simulink model "chris_3R_hsv_all_primitives_fixed_vortex"  (R2024b)
settings: Solver=FixedStepDiscrete  StartTime=0.0  StopTime=10  FixedStep=0.1  MaxStep=0.1  RelTol=1e-3
libraries: neural x102, realtime_pacer_lib x1, simulink x1
(part 6 of 6)

== matlab function chris_3R_hsv_all_primitives_fixed_vortex/all_bot_version2/sat_post_processor1 ==
  data: data output; data_raw input
function data = data_normalizing(data_raw)

data = (data_raw*2)-1;


end

== matlab function chris_3R_hsv_all_primitives_fixed_vortex/vector2scalar _avg_direction_only/Cluster Velocities to Cartesian Velocities ==
  data: fwdkin input; xc_err input; x1 output; zc_err input; thC_err input; a_err input; b_err input; C_err input; z1 output; th1 output; x2 output; z2 output; th2 output; x3 output; z3 output; th3 output
function [x1, z1,th1, x2,z2,th2, x3,z3, th3] = InverseJabobian(fwdkin, xc_err, zc_err, thC_err, a_err, b_err, C_err)
%% Unpacking the information from fwd_kin
p = fwdkin(1);
q = fwdkin(2);
beta = fwdkin(3);
xc = fwdkin(4);
yc = fwdkin(5);
theta_c = fwdkin(6);
yc_err = zc_err;
theta_c_err = thC_err;
p_err = a_err;
q_err = b_err;
beta_err = C_err;
%% Inverse Kinematics
  % Calculate x1, y1, and theta1 (Equations 12, 13, and 14)
r = sqrt((q + p*cos(beta))^2 + (p*sin(beta))^2);
  
x1 = xc + (1/3)*r*sin(theta_c);
y1 = yc + (1/3)*r*cos(theta_c);
%theta1 = phi1 - theta_c;
% Calculate x2, y2, and theta2 (Equations 15, 16, and 17)
x2 = xc + (1/3)*r*sin(theta_c) - p*sin(beta/2 + theta_c);
y2 = yc + (1/3)*r*cos(theta_c) - p*cos(beta/2 + theta_c);
%theta2 = phi2 - theta_c;
% Calculate x3, y3, and theta3 (Equations 18, 19, and 20)
x3 = xc + (1/3)*r*sin(theta_c) + q*sin(beta/2 - theta_c);
y3 = yc + (1/3)*r*cos(theta_c) - q*cos(beta/2 - theta_c);
%theta3 = phi3 - theta_c;
%% Now to take the partial derivates
% syms p q beta xc yc theta_c p_err q_err beta_err xc_err yc_err theta_c_err
% 
% % Define the equations
% eqs = [
%   xc + (1/3)*(sqrt((q + p*cos(beta))^2 + (p*sin(beta))^2))*sin(theta_c); % x1
%   yc + (1/3)*(sqrt((q + p*cos(beta))^2 + (p*sin(beta))^2))*cos(theta_c); % y1
%   xc + (1/3)*(sqrt((q + p*cos(beta))^2 + (p*sin(beta))^2))*sin(theta_c) - p*sin(beta/2 + theta_c); % x2
%   yc + (1/3)*(sqrt((q + p*cos(beta))^2 + (p*sin(beta))^2))*cos(theta_c) - p*cos(beta/2 + theta_c); % y2
%   xc + (1/3)*(sqrt((q + p*cos(beta))^2 + (p*sin(beta))^2))*sin(theta_c) + q*sin(beta/2 - theta_c); % x3
%   yc + (1/3)*(sqrt((q + p*cos(beta))^2 + (p*sin(beta))^2))*cos(theta_c) - q*cos(beta/2 - theta_c)  % y3
% ];
% 
% % Define the variables for differentiation
% vars = [p, q, beta, xc, yc, theta_c];
% 
% % Define the errors
% errs = [p_err, q_err, beta_err, xc_err, yc_err, theta_c_err];
% 
% % Initialize an array to store the sums (as symbolic)
% sums = sym(zeros(length(eqs), 1));
% 
% % Loop through equations and variables
% for i = 1:length(eqs)
%   for j = 1:length(vars)
%     derivative = diff(eqs(i), vars(j));
%     sums(i) = sums(i) + derivative * errs(j);
%   end
% end
% 
% % Display the results
% disp(simplify(sums(1)))
% disp(simplify(sums(2)))
% disp(simplify(sums(3)))
% disp(simplify(sums(4)))
% disp(simplify(sums(5)))
% disp(simplify(sums(6)))
%% Now to sum it all up
x1 =(3*xc_err*(p^2 + 2*cos(beta)*p*q + q^2)^(1/2) + p*p_err*sin(theta_c) + q*q_err*sin(theta_c) + p^2*theta_c_err*cos(theta_c) + q^2*theta_c_err*cos(theta_c) + p*q_err*cos(beta)*sin(theta_c) + p_err*q*cos(beta)*sin(theta_c) + 2*p*q*theta_c_err*cos(beta)*cos(theta_c) - beta_err*p*q*sin(beta)*sin(theta_c))/(3*(p^2 + 2*cos(beta)*p*q + q^2)^(1/2));
 
z1 = (3*yc_err*(p^2 + 2*cos(beta)*p*q + q^2)^(1/2) + p*p_err*cos(theta_c) + q*q_err*cos(theta_c) - p^2*theta_c_err*sin(theta_c) - q^2*theta_c_err*sin(theta_c) + p*q_err*cos(beta)*cos(theta_c) + p_err*q*cos(beta)*cos(theta_c) - beta_err*p*q*sin(beta)*cos(theta_c) - 2*p*q*theta_c_err*cos(beta)*sin(theta_c))/(3*(p^2 + 2*cos(beta)*p*q + q^2)^(1/2));
 
x2 = xc_err - p_err*(sin(beta/2 + theta_c) - (sin(theta_c)*(p + q*cos(beta)))/(3*(p^2 + 2*cos(beta)*p*q + q^2)^(1/2))) - beta_err*((p*cos(beta/2 + theta_c))/2 + (p*q*sin(beta)*sin(theta_c))/(3*(p^2 + 2*cos(beta)*p*q + q^2)^(1/2))) + theta_c_err*((cos(theta_c)*(p^2 + 2*cos(beta)*p*q + q^2)^(1/2))/3 - p*cos(beta/2 + theta_c)) + (q_err*sin(theta_c)*(q + p*cos(beta)))/(3*(p^2 + 2*cos(beta)*p*q + q^2)^(1/2));
 
z2 = yc_err - p_err*(cos(beta/2 + theta_c) - (cos(theta_c)*(p + q*cos(beta)))/(3*(p^2 + 2*cos(beta)*p*q + q^2)^(1/2))) + beta_err*((p*sin(beta/2 + theta_c))/2 - (p*q*sin(beta)*cos(theta_c))/(3*(p^2 + 2*cos(beta)*p*q + q^2)^(1/2))) - (theta_c_err*sin(theta_c)*(p^2 + 2*cos(beta)*p*q + q^2)^(1/2))/3 + p*theta_c_err*sin(beta/2 + theta_c) + (q_err*cos(theta_c)*(q + p*cos(beta)))/(3*(p^2 + 2*cos(beta)*p*q + q^2)^(1/2));
 
x3 = xc_err + q_err*(sin(beta/2 - theta_c) + (sin(theta_c)*(q + p*cos(beta)))/(3*(p^2 + 2*cos(beta)*p*q + q^2)^(1/2))) + beta_err*((q*cos(beta/2 - theta_c))/2 - (p*q*sin(beta)*sin(theta_c))/(3*(p^2 + 2*cos(beta)*p*q + q^2)^(1/2))) + (theta_c_err*cos(theta_c)*(p^2 + 2*cos(beta)*p*q + q^2)^(1/2))/3 - q*theta_c_err*cos(beta/2 - theta_c) + (p_err*sin(theta_c)*(p + q*cos(beta)))/(3*(p^2 + 2*cos(beta)*p*q + q^2)^(1/2));
 
z3 = yc_err - theta_c_err*(q*sin(beta/2 - theta_c) + (sin(theta_c)*(p^2 + 2*cos(beta)*p*q + q^2)^(1/2))/3) - q_err*(cos(beta/2 - theta_c) - (cos(theta_c)*(q + p*cos(beta)))/(3*(p^2 + 2*cos(beta)*p*q + q^2)^(1/2))) + beta_err*((q*sin(beta/2 - theta_c))/2 - (p*q*sin(beta)*cos(theta_c))/(3*(p^2 + 2*cos(beta)*p*q + q^2)^(1/2))) + (p_err*cos(theta_c)*(p + q*cos(beta)))/(3*(p^2 + 2*cos(beta)*p*q + q^2)^(1/2));
 
th1 = 0;
th2 = 0;
th3 = 0;

== matlab function chris_3R_hsv_all_primitives_fixed_vortex/Robot_signal_processing_3/Global to Body Rotation Matrix ==
  data: u input; y output
function y = fcn(u)

y = [cos(u) -sin(u) 0; sin(u) cos(u) 0; 0 0 1];

== matlab function chris_3R_hsv_all_primitives_fixed_vortex/Fixed_Vortex_Simulated_Environment/Fixed_Vortex_Simulator ==
  data: x input; hue_anticipated output; z input; sat_anticipated output; th input
function [hue_anticipated,sat_anticipated]= simulated_readings(x,z,th)

sat_anticipated = (((x^2 + z^2)^0.5)*.54) + 0.3;
hue_anticipated = atan2(z,x);

end

== matlab function chris_3R_hsv_all_primitives_fixed_vortex/Fixed_Vortex_Simulated_Environment/Fixed_Vortex_Simulator1 ==
  data: x input; hue_anticipated output; z input; sat_anticipated output; th input
function [hue_anticipated,sat_anticipated]= simulated_readings(x,z,th)

sat_anticipated = (((x^2 + z^2)^0.5)*.54) + 0.3;
hue_anticipated = atan2(z,x);

end

== matlab function chris_3R_hsv_all_primitives_fixed_vortex/Fixed_Vortex_Simulated_Environment/Fixed_Vortex_Simulator2 ==
  data: x input; hue_anticipated output; z input; sat_anticipated output; th input
function [hue_anticipated,sat_anticipated]= simulated_readings(x,z,th)

sat_anticipated = (((x^2 + z^2)^0.5)*.54) + 0.3;
hue_anticipated = atan2(z,x);

end

== matlab function chris_3R_hsv_all_primitives_fixed_vortex/vector2scalar_mag_steepest_descent/3_robot HSV to vector/MATLAB Function ==
  data: x output; x1 input; y output; y1 input; z1 input; x2 input; y2 input; z2 input; x3 input; y3 input; z3 input
function [x, y] = steepestDescent(x1, y1, z1, x2, y2, z2, x3, y3, z3)
  % Create vectors AB and AC
  AB = [x2 - x1, y2 - y1, z2 - z1];
  AC = [x3 - x1, y3 - y1, z3 - z1];

  % Calculate the cross product to get the normal vector
  N = cross(-AB, AC);

  % Get the direction of steepest descent (-N)
  descent =-N;

  % Normalize the vector to have unit length in the xy-plane
  magnitude = sqrt(descent(1)^2 + descent(2)^2);
  x = descent(1) / magnitude;
  y = descent(2) / magnitude;
  x = x/5;
  y = y/5;
end

== matlab function chris_3R_hsv_all_primitives_fixed_vortex/vector2scalar_mag_steepest_descent/Cartesian to Cluster Variables ==
  data: fwdkin output; x1 input; x_c output; y1 input; th1 input; x2 input; y2 input; th2 input; x3 input; y3 input; th3 input; y_c output; th_c output; a output; b output; c output; phi1 output; phi2 output; phi3 output
function [fwdkin, x_c, y_c, th_c, a, b, c,phi1,phi2,phi3]   = Forward_Kinematics(x1, y1, th1, x2,y2,th2, x3,y3,th3)
% Centre frame
x_c = (x1+x2+x3)/3;
y_c = (y1+y2+y3)/3;
theta_c = atan2((2/3)*x1 - (1/3)*(x2 + x3), (2/3)*y1 - (1/3)*(y2 + y3));
% SAS Properties of triangle
p = sqrt((x1 - x2)^2 + (y1 - y2)^2);
q = sqrt((x3 - x1)^2 + (y1 - y3)^2);
beta = acos((p^2 + q^2 - (x3 - x2)^2 - (y3 - y2)^2) / (2*p*q));
% Rotation vectors
phi1 = th1 + theta_c;
phi2 = th2 + theta_c;
phi3 = th3 + theta_c;
a =p;
b = q;
c = beta;
th_c = theta_c;
fwdkin = [0 0 0 0 0 0];
fwdkin(1) =a;
fwdkin(2) =b;
fwdkin(3) =c;
fwdkin(4) =x_c;
fwdkin(5) =y_c;
fwdkin(6) =th_c;

== matlab function chris_3R_hsv_all_primitives_fixed_vortex/Cluster_Controller_setpoint/Cartesian to Cluster Variables ==
  data: fwdkin output; x1 input; x_c output; y1 input; th1 input; x2 input; y2 input; th2 input; x3 input; y3 input; th3 input; y_c output; th_c output; a output; b output; c output
function [fwdkin, x_c, y_c, th_c, a, b, c]   = Forward_Kinematics(x1, y1, th1, x2,y2,th2, x3,y3,th3)
% Centre frame
x_c = (x1+x2+x3)/3;
y_c = (y1+y2+y3)/3;
theta_c = atan2((2/3)*x1 - (1/3)*(x2 + x3), (2/3)*y1 - (1/3)*(y2 + y3));
% SAS Properties of triangle
p = sqrt((x1 - x2)^2 + (y1 - y2)^2);
q = sqrt((x3 - x1)^2 + (y1 - y3)^2);
beta = acos((p^2 + q^2 - (x3 - x2)^2 - (y3 - y2)^2) / (2*p*q));
% Rotation vectors
phi1 = th1 + theta_c;
phi2 = th2 + theta_c;
phi3 = th3 + theta_c;
a =p;
b = q;
c = beta;
th_c = theta_c;
fwdkin = [0 0 0 0 0 0];
fwdkin(1) =a;
fwdkin(2) =b;
fwdkin(3) =c;
fwdkin(4) =x_c;
fwdkin(5) =y_c;
fwdkin(6) =th_c;

== matlab function chris_3R_hsv_all_primitives_fixed_vortex/vector2scalar_mag_steepest_descent/Cluster Velocities to Cartesian Velocities ==
  data: fwdkin input; xc_err input; x1 output; zc_err input; thC_err input; a_err input; b_err input; C_err input; z1 output; th1 output; x2 output; z2 output; th2 output; x3 output; z3 output; th3 output
function [x1, z1,th1, x2,z2,th2, x3,z3, th3] = InverseJabobian(fwdkin, xc_err, zc_err, thC_err, a_err, b_err, C_err)
%% Unpacking the information from fwd_kin
p = fwdkin(1);
q = fwdkin(2);
beta = fwdkin(3);
xc = fwdkin(4);
yc = fwdkin(5);
theta_c = fwdkin(6);
yc_err = zc_err;
theta_c_err = thC_err;
p_err = a_err;
q_err = b_err;
beta_err = C_err;
%% Inverse Kinematics
  % Calculate x1, y1, and theta1 (Equations 12, 13, and 14)
r = sqrt((q + p*cos(beta))^2 + (p*sin(beta))^2);
  
x1 = xc + (1/3)*r*sin(theta_c);
y1 = yc + (1/3)*r*cos(theta_c);
%theta1 = phi1 - theta_c;
% Calculate x2, y2, and theta2 (Equations 15, 16, and 17)
x2 = xc + (1/3)*r*sin(theta_c) - p*sin(beta/2 + theta_c);
y2 = yc + (1/3)*r*cos(theta_c) - p*cos(beta/2 + theta_c);
%theta2 = phi2 - theta_c;
% Calculate x3, y3, and theta3 (Equations 18, 19, and 20)
x3 = xc + (1/3)*r*sin(theta_c) + q*sin(beta/2 - theta_c);
y3 = yc + (1/3)*r*cos(theta_c) - q*cos(beta/2 - theta_c);
%theta3 = phi3 - theta_c;
%% Now to take the partial derivates
% syms p q beta xc yc theta_c p_err q_err beta_err xc_err yc_err theta_c_err
% 
% % Define the equations
% eqs = [
%   xc + (1/3)*(sqrt((q + p*cos(beta))^2 + (p*sin(beta))^2))*sin(theta_c); % x1
%   yc + (1/3)*(sqrt((q + p*cos(beta))^2 + (p*sin(beta))^2))*cos(theta_c); % y1
%   xc + (1/3)*(sqrt((q + p*cos(beta))^2 + (p*sin(beta))^2))*sin(theta_c) - p*sin(beta/2 + theta_c); % x2
%   yc + (1/3)*(sqrt((q + p*cos(beta))^2 + (p*sin(beta))^2))*cos(theta_c) - p*cos(beta/2 + theta_c); % y2
%   xc + (1/3)*(sqrt((q + p*cos(beta))^2 + (p*sin(beta))^2))*sin(theta_c) + q*sin(beta/2 - theta_c); % x3
%   yc + (1/3)*(sqrt((q + p*cos(beta))^2 + (p*sin(beta))^2))*cos(theta_c) - q*cos(beta/2 - theta_c)  % y3
% ];
% 
% % Define the variables for differentiation
% vars = [p, q, beta, xc, yc, theta_c];
% 
% % Define the errors
% errs = [p_err, q_err, beta_err, xc_err, yc_err, theta_c_err];
% 
% % Initialize an array to store the sums (as symbolic)
% sums = sym(zeros(length(eqs), 1));
% 
% % Loop through equations and variables
% for i = 1:length(eqs)
%   for j = 1:length(vars)
%     derivative = diff(eqs(i), vars(j));
%     sums(i) = sums(i) + derivative * errs(j);
%   end
% end
% 
% % Display the results
% disp(simplify(sums(1)))
% disp(simplify(sums(2)))
% disp(simplify(sums(3)))
% disp(simplify(sums(4)))
% disp(simplify(sums(5)))
% disp(simplify(sums(6)))
%% Now to sum it all up
x1 =(3*xc_err*(p^2 + 2*cos(beta)*p*q + q^2)^(1/2) + p*p_err*sin(theta_c) + q*q_err*sin(theta_c) + p^2*theta_c_err*cos(theta_c) + q^2*theta_c_err*cos(theta_c) + p*q_err*cos(beta)*sin(theta_c) + p_err*q*cos(beta)*sin(theta_c) + 2*p*q*theta_c_err*cos(beta)*cos(theta_c) - beta_err*p*q*sin(beta)*sin(theta_c))/(3*(p^2 + 2*cos(beta)*p*q + q^2)^(1/2));
 
z1 = (3*yc_err*(p^2 + 2*cos(beta)*p*q + q^2)^(1/2) + p*p_err*cos(theta_c) + q*q_err*cos(theta_c) - p^2*theta_c_err*sin(theta_c) - q^2*theta_c_err*sin(theta_c) + p*q_err*cos(beta)*cos(theta_c) + p_err*q*cos(beta)*cos(theta_c) - beta_err*p*q*sin(beta)*cos(theta_c) - 2*p*q*theta_c_err*cos(beta)*sin(theta_c))/(3*(p^2 + 2*cos(beta)*p*q + q^2)^(1/2));
 
x2 = xc_err - p_err*(sin(beta/2 + theta_c) - (sin(theta_c)*(p + q*cos(beta)))/(3*(p^2 + 2*cos(beta)*p*q + q^2)^(1/2))) - beta_err*((p*cos(beta/2 + theta_c))/2 + (p*q*sin(beta)*sin(theta_c))/(3*(p^2 + 2*cos(beta)*p*q + q^2)^(1/2))) + theta_c_err*((cos(theta_c)*(p^2 + 2*cos(beta)*p*q + q^2)^(1/2))/3 - p*cos(beta/2 + theta_c)) + (q_err*sin(theta_c)*(q + p*cos(beta)))/(3*(p^2 + 2*cos(beta)*p*q + q^2)^(1/2));
 
z2 = yc_err - p_err*(cos(beta/2 + theta_c) - (cos(theta_c)*(p + q*cos(beta)))/(3*(p^2 + 2*cos(beta)*p*q + q^2)^(1/2))) + beta_err*((p*sin(beta/2 + theta_c))/2 - (p*q*sin(beta)*cos(theta_c))/(3*(p^2 + 2*cos(beta)*p*q + q^2)^(1/2))) - (theta_c_err*sin(theta_c)*(p^2 + 2*cos(beta)*p*q + q^2)^(1/2))/3 + p*theta_c_err*sin(beta/2 + theta_c) + (q_err*cos(theta_c)*(q + p*cos(beta)))/(3*(p^2 + 2*cos(beta)*p*q + q^2)^(1/2));
 
x3 = xc_err + q_err*(sin(beta/2 - theta_c) + (sin(theta_c)*(q + p*cos(beta)))/(3*(p^2 + 2*cos(beta)*p*q + q^2)^(1/2))) + beta_err*((q*cos(beta/2 - theta_c))/2 - (p*q*sin(beta)*sin(theta_c))/(3*(p^2 + 2*cos(beta)*p*q + q^2)^(1/2))) + (theta_c_err*cos(theta_c)*(p^2 + 2*cos(beta)*p*q + q^2)^(1/2))/3 - q*theta_c_err*cos(beta/2 - theta_c) + (p_err*sin(theta_c)*(p + q*cos(beta)))/(3*(p^2 + 2*cos(beta)*p*q + q^2)^(1/2));
 
z3 = yc_err - theta_c_err*(q*sin(beta/2 - theta_c) + (sin(theta_c)*(p^2 + 2*cos(beta)*p*q + q^2)^(1/2))/3) - q_err*(cos(beta/2 - theta_c) - (cos(theta_c)*(q + p*cos(beta)))/(3*(p^2 + 2*cos(beta)*p*q + q^2)^(1/2))) + beta_err*((q*sin(beta/2 - theta_c))/2 - (p*q*sin(beta)*cos(theta_c))/(3*(p^2 + 2*cos(beta)*p*q + q^2)^(1/2))) + (p_err*cos(theta_c)*(p + q*cos(beta)))/(3*(p^2 + 2*cos(beta)*p*q + q^2)^(1/2));
 
th1 = 0;
th2 = 0;
th3 = 0;

== matlab function chris_3R_hsv_all_primitives_fixed_vortex/Cluster_Controller_setpoint/Cluster Velocities to Cartesian Velocities ==
  data: fwdkin input; xc_err input; x1 output; zc_err input; thC_err input; a_err input; b_err input; C_err input; z1 output; th1 output; x2 output; z2 output; th2 output; x3 output; z3 output; th3 output
function [x1, z1,th1, x2,z2,th2, x3,z3, th3] = InverseJabobian(fwdkin, xc_err, zc_err, thC_err, a_err, b_err, C_err)
%% Unpacking the information from fwd_kin
p = fwdkin(1);
q = fwdkin(2);
beta = fwdkin(3);
xc = fwdkin(4);
yc = fwdkin(5);
theta_c = fwdkin(6);
yc_err = zc_err;
theta_c_err = thC_err;
p_err = a_err;
q_err = b_err;
beta_err = C_err;
%% Inverse Kinematics
  % Calculate x1, y1, and theta1 (Equations 12, 13, and 14)
r = sqrt((q + p*cos(beta))^2 + (p*sin(beta))^2);
  
x1 = xc + (1/3)*r*sin(theta_c);
y1 = yc + (1/3)*r*cos(theta_c);
%theta1 = phi1 - theta_c;
% Calculate x2, y2, and theta2 (Equations 15, 16, and 17)
x2 = xc + (1/3)*r*sin(theta_c) - p*sin(beta/2 + theta_c);
y2 = yc + (1/3)*r*cos(theta_c) - p*cos(beta/2 + theta_c);
%theta2 = phi2 - theta_c;
% Calculate x3, y3, and theta3 (Equations 18, 19, and 20)
x3 = xc + (1/3)*r*sin(theta_c) + q*sin(beta/2 - theta_c);
y3 = yc + (1/3)*r*cos(theta_c) - q*cos(beta/2 - theta_c);
%theta3 = phi3 - theta_c;
%% Now to take the partial derivates
% syms p q beta xc yc theta_c p_err q_err beta_err xc_err yc_err theta_c_err
% 
% % Define the equations
% eqs = [
%   xc + (1/3)*(sqrt((q + p*cos(beta))^2 + (p*sin(beta))^2))*sin(theta_c); % x1
%   yc + (1/3)*(sqrt((q + p*cos(beta))^2 + (p*sin(beta))^2))*cos(theta_c); % y1
%   xc + (1/3)*(sqrt((q + p*cos(beta))^2 + (p*sin(beta))^2))*sin(theta_c) - p*sin(beta/2 + theta_c); % x2
%   yc + (1/3)*(sqrt((q + p*cos(beta))^2 + (p*sin(beta))^2))*cos(theta_c) - p*cos(beta/2 + theta_c); % y2
%   xc + (1/3)*(sqrt((q + p*cos(beta))^2 + (p*sin(beta))^2))*sin(theta_c) + q*sin(beta/2 - theta_c); % x3
%   yc + (1/3)*(sqrt((q + p*cos(beta))^2 + (p*sin(beta))^2))*cos(theta_c) - q*cos(beta/2 - theta_c)  % y3
% ];
% 
% % Define the variables for differentiation
% vars = [p, q, beta, xc, yc, theta_c];
% 
% % Define the errors
% errs = [p_err, q_err, beta_err, xc_err, yc_err, theta_c_err];
% 
% % Initialize an array to store the sums (as symbolic)
% sums = sym(zeros(length(eqs), 1));
% 
% % Loop through equations and variables
% for i = 1:length(eqs)
%   for j = 1:length(vars)
%     derivative = diff(eqs(i), vars(j));
%     sums(i) = sums(i) + derivative * errs(j);
%   end
% end
% 
% % Display the results
% disp(simplify(sums(1)))
% disp(simplify(sums(2)))
% disp(simplify(sums(3)))
% disp(simplify(sums(4)))
% disp(simplify(sums(5)))
% disp(simplify(sums(6)))
%% Now to sum it all up
x1 =(3*xc_err*(p^2 + 2*cos(beta)*p*q + q^2)^(1/2) + p*p_err*sin(theta_c) + q*q_err*sin(theta_c) + p^2*theta_c_err*cos(theta_c) + q^2*theta_c_err*cos(theta_c) + p*q_err*cos(beta)*sin(theta_c) + p_err*q*cos(beta)*sin(theta_c) + 2*p*q*theta_c_err*cos(beta)*cos(theta_c) - beta_err*p*q*sin(beta)*sin(theta_c))/(3*(p^2 + 2*cos(beta)*p*q + q^2)^(1/2));
 
z1 = (3*yc_err*(p^2 + 2*cos(beta)*p*q + q^2)^(1/2) + p*p_err*cos(theta_c) + q*q_err*cos(theta_c) - p^2*theta_c_err*sin(theta_c) - q^2*theta_c_err*sin(theta_c) + p*q_err*cos(beta)*cos(theta_c) + p_err*q*cos(beta)*cos(theta_c) - beta_err*p*q*sin(beta)*cos(theta_c) - 2*p*q*theta_c_err*cos(beta)*sin(theta_c))/(3*(p^2 + 2*cos(beta)*p*q + q^2)^(1/2));
 
x2 = xc_err - p_err*(sin(beta/2 + theta_c) - (sin(theta_c)*(p + q*cos(beta)))/(3*(p^2 + 2*cos(beta)*p*q + q^2)^(1/2))) - beta_err*((p*cos(beta/2 + theta_c))/2 + (p*q*sin(beta)*sin(theta_c))/(3*(p^2 + 2*cos(beta)*p*q + q^2)^(1/2))) + theta_c_err*((cos(theta_c)*(p^2 + 2*cos(beta)*p*q + q^2)^(1/2))/3 - p*cos(beta/2 + theta_c)) + (q_err*sin(theta_c)*(q + p*cos(beta)))/(3*(p^2 + 2*cos(beta)*p*q + q^2)^(1/2));
 
z2 = yc_err - p_err*(cos(beta/2 + theta_c) - (cos(theta_c)*(p + q*cos(beta)))/(3*(p^2 + 2*cos(beta)*p*q + q^2)^(1/2))) + beta_err*((p*sin(beta/2 + theta_c))/2 - (p*q*sin(beta)*cos(theta_c))/(3*(p^2 + 2*cos(beta)*p*q + q^2)^(1/2))) - (theta_c_err*sin(theta_c)*(p^2 + 2*cos(beta)*p*q + q^2)^(1/2))/3 + p*theta_c_err*sin(beta/2 + theta_c) + (q_err*cos(theta_c)*(q + p*cos(beta)))/(3*(p^2 + 2*cos(beta)*p*q + q^2)^(1/2));
 
x3 = xc_err + q_err*(sin(beta/2 - theta_c) + (sin(theta_c)*(q + p*cos(beta)))/(3*(p^2 + 2*cos(beta)*p*q + q^2)^(1/2))) + beta_err*((q*cos(beta/2 - theta_c))/2 - (p*q*sin(beta)*sin(theta_c))/(3*(p^2 + 2*cos(beta)*p*q + q^2)^(1/2))) + (theta_c_err*cos(theta_c)*(p^2 + 2*cos(beta)*p*q + q^2)^(1/2))/3 - q*theta_c_err*cos(beta/2 - theta_c) + (p_err*sin(theta_c)*(p + q*cos(beta)))/(3*(p^2 + 2*cos(beta)*p*q + q^2)^(1/2));
 
z3 = yc_err - theta_c_err*(q*sin(beta/2 - theta_c) + (sin(theta_c)*(p^2 + 2*cos(beta)*p*q + q^2)^(1/2))/3) - q_err*(cos(beta/2 - theta_c) - (cos(theta_c)*(q + p*cos(beta)))/(3*(p^2 + 2*cos(beta)*p*q + q^2)^(1/2))) + beta_err*((q*sin(beta/2 - theta_c))/2 - (p*q*sin(beta)*cos(theta_c))/(3*(p^2 + 2*cos(beta)*p*q + q^2)^(1/2))) + (p_err*cos(theta_c)*(p + q*cos(beta)))/(3*(p^2 + 2*cos(beta)*p*q + q^2)^(1/2));
 
th1 = 0;
th2 = 0;
th3 = 0;

== matlab function chris_3R_hsv_all_primitives_fixed_vortex/Robot_signal_processing_1/Global to Body Rotation Matrix ==
  data: u input; y output
function y = fcn(u)

y = [cos(u) -sin(u) 0; sin(u) cos(u) 0; 0 0 1];

== matlab function chris_3R_hsv_all_primitives_fixed_vortex/FullVector_VectorSum/Cartesian to Cluster Variables ==
  data: fwdkin output; x1 input; x_c output; y1 input; th1 input; x2 input; y2 input; th2 input; x3 input; y3 input; th3 input; y_c output; th_c output; a output; b output; c output
function [fwdkin, x_c, y_c, th_c, a, b, c]   = Forward_Kinematics(x1, y1, th1, x2,y2,th2, x3,y3,th3)
% Centre frame
x_c = (x1+x2+x3)/3;
y_c = (y1+y2+y3)/3;
theta_c = atan2((2/3)*x1 - (1/3)*(x2 + x3), (2/3)*y1 - (1/3)*(y2 + y3));
% SAS Properties of triangle
p = sqrt((x1 - x2)^2 + (y1 - y2)^2);
q = sqrt((x3 - x1)^2 + (y1 - y3)^2);
beta = acos((p^2 + q^2 - (x3 - x2)^2 - (y3 - y2)^2) / (2*p*q));
% Rotation vectors
phi1 = th1 + theta_c;
phi2 = th2 + theta_c;
phi3 = th3 + theta_c;
a =p;
b = q;
c = beta;
th_c = theta_c;
fwdkin = [0 0 0 0 0 0];
fwdkin(1) =a;
fwdkin(2) =b;
fwdkin(3) =c;
fwdkin(4) =x_c;
fwdkin(5) =y_c;
fwdkin(6) =th_c;
